simulink model "Task_4_Signal"  (R2025a)
settings: Solver=ode4  StartTime=0.0  StopTime=2  FixedStep=0.00001  RelTol=1e-3
model workspace (MAT data in the model file):
  C = 50
  K = 75
  StartDist = 0.2
  V = 3
  m = 10
libraries: simulink x3
settings Model: Creator=jmorc  LastModifiedBy=henri

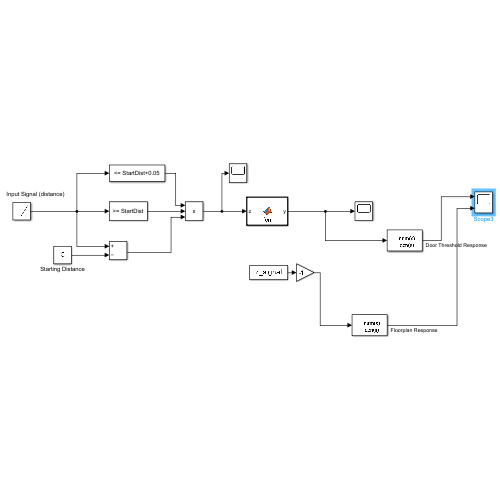
[thumbnail: Simulink's stored preview of the top-level diagram]
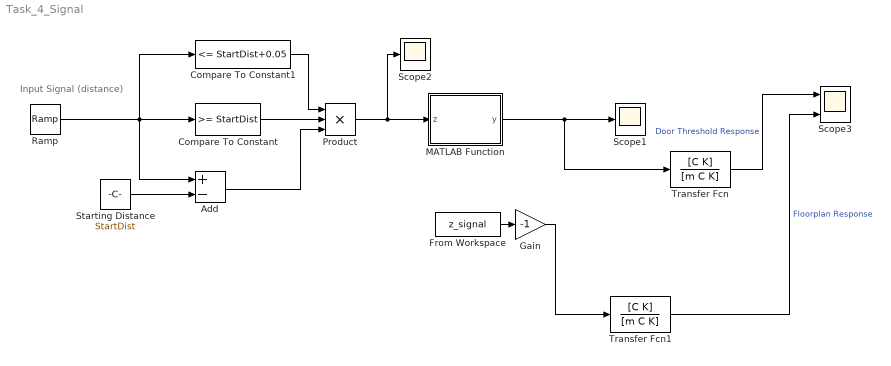
== system Task_4_Signal ==
  note: Input Signal (distance)
  Add : Sum  Inputs=+-
  Compare To Constant : simulink/Logic and Bit Operations/Compare To Constant  relop=>=  const=StartDist  OutDataTypeStr=boolean
  Compare To Constant1 : simulink/Logic and Bit Operations/Compare To Constant  relop=<=  const=StartDist+0.05  OutDataTypeStr=boolean
  From Workspace : FromWorkspace  VariableName=z_signal  OutputAfterFinalValue=Holding final value
  Gain : Gain  Gain=-1
  MATLAB Function : MATLAB Function  TreatAsAtomicUnit=on
  Product : Product  Inputs=3
  Ramp : simulink/Sources/Ramp  slope=1  start=0  InitialOutput=0
  Scope1 : Scope
      settings: ActiveDisplayYMinimum=-0.016249587732509282  ActiveDisplayYMaximum=0.075321611313754436
  Scope2 : Scope
      settings: ActiveDisplayYMinimum=-0.012589931548242353  ActiveDisplayYMaximum=0.08436808195041462  DataLoggingVariableName=ScopeData2
  Scope3 : Scope  NumInputPorts=2
      settings: ActiveDisplayYMinimum=-0.00057159990857951414  ActiveDisplayYMaximum=0.0039217521977168617  YLabel=Vertical Displacement (m)  DataLoggingVariableName=ScopeData3
  Starting Distance : Constant  Value=StartDist
  Transfer Fcn : TransferFcn  Numerator=[C K]  Denominator=[m C K]
  Transfer Fcn1 : TransferFcn  Numerator=[C K]  Denominator=[m C K]
  wires:
  Ramp/1 -> Compare To Constant1/1, Add/1, Compare To Constant/1
  Starting Distance/1 -> Add/2
  Compare To Constant/1 -> Product/2
  Add/1 -> Product/3
  Compare To Constant1/1 -> Product/1
  Product/1 -> Scope2/1, MATLAB Function/1(z)
  Transfer Fcn/1 -> Scope3/1  "Door Threshold Response"
  MATLAB Function/1(y) -> Transfer Fcn/1, Scope1/1
  From Workspace/1 -> Gain/1
  Gain/1 -> Transfer Fcn1/1
  Transfer Fcn1/1 -> Scope3/2  "Floorplan Response"

== matlab function Task_4_Signal/MATLAB Function ==
  data: z input; y output
function y = fcn(z)
    y = 0.03 * sin(pi * z / 0.05)^2;
end
